simulink model "Discretisation_AleixGranero_MichalSzabo"  (R2021b)
settings: Solver=ode3  StartTime=0.0  StopTime=1000  FixedStep=Ts  RelTol=1e-3  EnableMultiTasking=on
values from neighbouring files (symbols this model uses):
  A = [K1   0 -K3   0 ... (first row only)    [Discretisation_MichalSzabo_AleixGranero.m]    (also in Linearisation_MichalSzabo_AleixGranero.m)
  alpha = - 0.5 * (a1/A1) * (1/sqrt(2*g*h10)) * 2 * g    [Discretisation_MichalSzabo_AleixGranero.m]
  B = [J2 0 ... (first row only)    [Discretisation_MichalSzabo_AleixGranero.m]    (also in Linearisation_MichalSzabo_AleixGranero.m)
  beta = 0.5 * (a3/A1) * (1/sqrt(2*g*h30)) * 2 * g    [Discretisation_MichalSzabo_AleixGranero.m]
  C = eye(4)    [Discretisation_MichalSzabo_AleixGranero.m]    (also in Linearisation_MichalSzabo_AleixGranero.m)
  D = zeros(4,2)    [Discretisation_MichalSzabo_AleixGranero.m]    (also in Linearisation_MichalSzabo_AleixGranero.m)
  h10 = 1/(2*g)*(a3/a1 * sqrt(2*g*h30)+gamma1*k1/a1*v10)^2    [Discretisation_MichalSzabo_AleixGranero.m]    (also in Linearisation_MichalSzabo_AleixGranero.m)
  h20 = 1/(2*g)*(a4/a2 * sqrt(2*g*h40)+gamma2*k1/a2*v20)^2    [Discretisation_MichalSzabo_AleixGranero.m]    (also in Linearisation_MichalSzabo_AleixGranero.m)
  h30 = 1/(2*g)*((1-gamma2)*k2*v20/a3)^2    (= 0.40362240636)    [Discretisation_MichalSzabo_AleixGranero.m]    (also in Linearisation_MichalSzabo_AleixGranero.m)
  h40 = 1/(2*g)*((1-gamma1)*k2*v10/a4)^2    (= 0.40362240636)    [Discretisation_MichalSzabo_AleixGranero.m]    (also in Linearisation_MichalSzabo_AleixGranero.m)
  omega = gamma1 * k1/A1    (= 0.08325)    [Discretisation_MichalSzabo_AleixGranero.m]
  t1 = 200    [Discretisation_MichalSzabo_AleixGranero.m]    (also in Linearisation_MichalSzabo_AleixGranero.m)
  t2 = 400    [Discretisation_MichalSzabo_AleixGranero.m]    (also in Linearisation_MichalSzabo_AleixGranero.m)
  v10 = 2    [Discretisation_MichalSzabo_AleixGranero.m]    (also in Linearisation_MichalSzabo_AleixGranero.m)
  v11 = 2.2    [Discretisation_MichalSzabo_AleixGranero.m]    (also in Linearisation_MichalSzabo_AleixGranero.m)
  v20 = 2    [Discretisation_MichalSzabo_AleixGranero.m]    (also in Linearisation_MichalSzabo_AleixGranero.m)
  v22 = 1.8    [Discretisation_MichalSzabo_AleixGranero.m]    (also in Linearisation_MichalSzabo_AleixGranero.m)
settings Model: Creator=as  LastModifiedBy=szmis
settings SolverCC: AlgebraicLoopSolver=TrustRegion
settings DataIOCC: LimitDataPoints=on  SaveFormat=Array  SignalLoggingSaveFormat=ModelDataLogs  ReturnWorkspaceOutputs=off
settings OptimizationCC: LifeSpan=inf
settings DebuggingCC: SaveWithParameterizedLinksMsg=none  UnderspecifiedInitializationDetection=Classic  MergeDetectMultiDrivingBlocksExec=none  SolverPrmCheckMsg=warning  FcnCallInpInsideContextMsg=warning  SFUnexpectedBacktrackingDiag=warning  SFNoUnconditionalDefaultTransitionDiag=warning  SFExecutionAtInitializationDiag=none  SFMachineParentedDataDiag=warning  ArithmeticOperatorsInVariantConditions=warning
settings HardwareCC: ProdBitPerPointer=32  ProdBitPerSizeT=32  ProdBitPerPtrDiffT=32  ProdLargestAtomicFloat=None  ProdIntDivRoundTo=Undefined  ProdEndianess=Unspecified  ProdWordSize=32  ProdHWDeviceType=32-bit Generic
settings ModelReferenceCC: PropagateSignalLabelsOutOfModel=off
settings SFSimCC: SimUseLocalCustomCode=off  CustomCodeUndefinedFunction=UseInterfaceOnly
settings RTWCC: RTWUseLocalCustomCode=off
settings CodeAppCC: StateflowObjectComments=on
settings GRTTargetCC: TargetLangStandard=C89/C90 (ANSI)  CombineOutputUpdateFcns=off  GRTInterface=on
settings ConfigComp: CovMetricSettings=dw  CovSaveCumulativeToWorkspaceVar=on  CovSaveSingleToWorkspaceVar=on  CovExternalEMLEnable=off

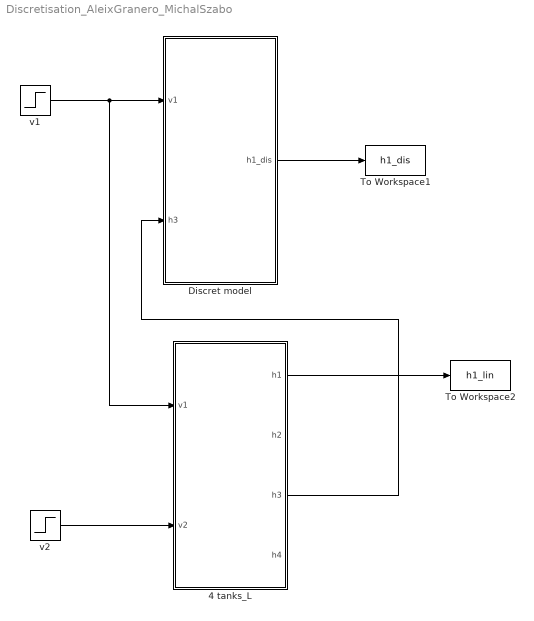
== system Discretisation_AleixGranero_MichalSzabo ==
  4 tanks_L : Subsystem
  Discret model : Subsystem
  To Workspace1 : ToWorkspace  VariableName=h1_dis  SampleTime=-1
  To Workspace2 : ToWorkspace  VariableName=h1_lin  SampleTime=-1
  v1 : Step  Time=t1  Before=v10  After=v11  SampleTime=0
  v2 : Step  Time=t2  Before=v20  After=v22  SampleTime=0
  wires:
  v1/1 -> 4 tanks_L/1(v1), Discret model/1(v1)
  4 tanks_L/1("h1 ") -> To Workspace2/1
  Discret model/1("h1_dis ") -> To Workspace1/1
  4 tanks_L/3("h3 ") -> Discret model/2(h3)
  v2/1 -> 4 tanks_L/2(v2)

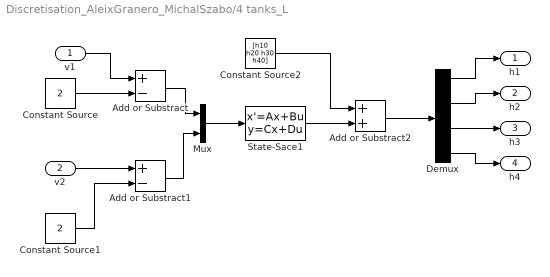
== system Discretisation_AleixGranero_MichalSzabo/4 tanks_L ==
  v1 : Inport
  v2 : Inport  Port=2
  Add or Substract : Sum  Inputs=+-
  Add or Substract1 : Sum  Inputs=+-
  Add or Substract2 : Sum
  Constant Source : Constant  Value=2
  Constant Source1 : Constant  Value=2
  Constant Source2 : Constant  Value=[h10 h20 h30 h40]
  Demux : Demux
  Mux : Mux  Inputs=2
  State-Sace1 : StateSpace  A=A  B=B  C=C  D=D  InitialCondition=0
  "h1 " : Outport
  "h2 " : Outport  Port=2
  "h3 " : Outport  Port=3
  "h4 " : Outport  Port=4
  wires:
  Mux/1 -> State-Sace1/1
  Constant Source/1 -> Add or Substract/2
  v1/1 -> Add or Substract/1
  v2/1 -> Add or Substract1/1
  Constant Source1/1 -> Add or Substract1/2
  Add or Substract/1 -> Mux/1
  Add or Substract1/1 -> Mux/2
  State-Sace1/1 -> Add or Substract2/2
  Add or Substract2/1 -> Demux/1
  Demux/1 -> "h1 "/1
  Demux/2 -> "h2 "/1
  Demux/3 -> "h3 "/1
  Demux/4 -> "h4 "/1
  Constant Source2/1 -> Add or Substract2/1

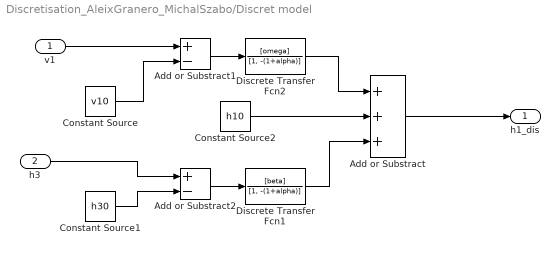
== system Discretisation_AleixGranero_MichalSzabo/Discret model ==
  v1 : Inport
  h3 : Inport  Port=2
  Add or Substract : Sum  Inputs=+++
  Add or Substract1 : Sum  Inputs=+-
  Add or Substract2 : Sum  Inputs=+-
  Constant Source : Constant  Value=v10
  Constant Source1 : Constant  Value=h30
  Constant Source2 : Constant  Value=h10
  Discrete Transfer Fcn1 : DiscreteTransferFcn  Numerator=[beta]  Denominator=[1, -(1+alpha)]  SampleTime=1
  Discrete Transfer Fcn2 : DiscreteTransferFcn  Numerator=[omega]  Denominator=[1, -(1+alpha)]  SampleTime=1
  "h1_dis " : Outport
  wires:
  Add or Substract/1 -> "h1_dis "/1
  v1/1 -> Add or Substract1/1
  h3/1 -> Add or Substract2/1
  Constant Source1/1 -> Add or Substract2/2
  Constant Source/1 -> Add or Substract1/2
  Constant Source2/1 -> Add or Substract/2
  Add or Substract1/1 -> Discrete Transfer Fcn2/1
  Add or Substract2/1 -> Discrete Transfer Fcn1/1
  Discrete Transfer Fcn2/1 -> Add or Substract/1
  Discrete Transfer Fcn1/1 -> Add or Substract/3
